simulink model "M12_addBlox"  (R2021a)
settings: Solver=ode45  StartTime=0.0  StopTime=10.0  RelTol=1e-3  EnableMultiTasking=on
undefined symbols (not defined in the file): magnitude, Tbit5_0
libraries: dspstat3 x4, simulink_extras x1, GeneralASKLib x1, commsink2 x1, NoiseLib_2021 x1
settings Model: Creator=Bornitz  LastModifiedBy=Bornitz
settings SolverCC: AlgebraicLoopSolver=TrustRegion
settings DataIOCC: LimitDataPoints=on  SaveFormat=Array
settings OptimizationCC: ExpressionDepthLimit=2147483647  LifeSpan=inf
settings DebuggingCC: SolverPrmCheckMsg=warning  StateNameClashWarn=warning  StrictBusMsg=ErrorOnBusTreatedAsVector  SFUnexpectedBacktrackingDiag=warning  SFNoUnconditionalDefaultTransitionDiag=warning  SFMachineParentedDataDiag=warning  ArithmeticOperatorsInVariantConditions=warning
settings HardwareCC: ProdBitPerPointer=32  ProdBitPerSizeT=32  ProdBitPerPtrDiffT=32  ProdLargestAtomicFloat=None  ProdIntDivRoundTo=Undefined  ProdEndianess=Unspecified  ProdWordSize=32  ProdHWDeviceType=32-bit Generic
settings ModelReferenceCC: PropagateSignalLabelsOutOfModel=off
settings SFSimCC: SimUseLocalCustomCode=off  SimParseCustomCode=off  CustomCodeUndefinedFunction=UseInterfaceOnly
settings RTWCC: RTWUseLocalCustomCode=off
settings CodeAppCC: StateflowObjectComments=on
settings GRTTargetCC: TargetLangStandard=C89/C90 (ANSI)  CombineOutputUpdateFcns=off  GRTInterface=on
settings ConfigComp: CovMetricSettings=dw  CovSaveCumulativeToWorkspaceVar=on  CovSaveSingleToWorkspaceVar=on  CovExternalEMLEnable=off  CovSFcnEnable=off

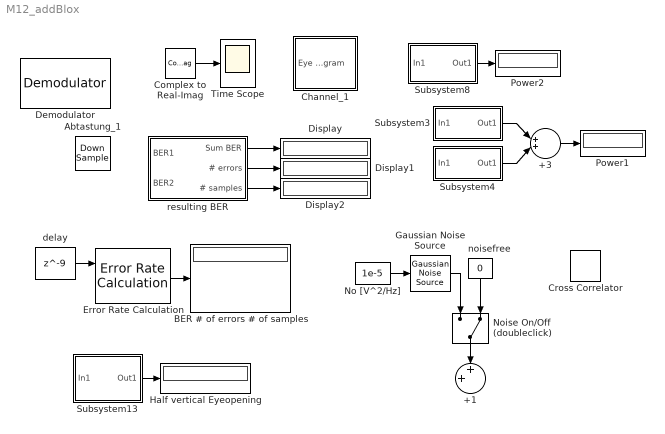
== system M12_addBlox ==
  " Power1" : Display
  " Power2" : Display
  +1 : Sum  Inputs=++|  SampleTime=Tbit5_0/16
  +3 : Sum  Inputs=||++||
  Abtastung_1 : DownSample  N=16  RateOptions=Allow multirate processing
  BER # of errors # of samples : Display
      settings: Format=short_e  Decimation=2
  Channel_1 : Subsystem
  Complex to Real-Imag : ComplexToRealImag  Output=Real
  Cross Correlator : simulink_extras/Additional Sinks/Cross Correlator  npts=100  HowOften=50  sampleT=0.0002
      settings: SourceProductBaseCode=SL
  Demodulator : GeneralASKLib/Demodulator  SystemSampleTime=-1  VariantActivationTime=update diagram  Latency=0  AutoFrameSizeCalculation=off
  Display : Display
      settings: Format=short_e
  Display1 : Display
  Display2 : Display
  Error Rate Calculation : commsink2/Error Rate Calculation  N=0  st_delay=100  cp_mode=Entire frame  subframe=1  PMode=Port  WsName=ErrorVec  RsMode2=off  stop=off  numErr=100  maxBits=1e6
  Gaussian Noise Source : NoiseLib_2021/Gaussian Noise Source  SystemSampleTime=-1  VariantActivationTime=update diagram  Latency=0  AutoFrameSizeCalculation=off
  Half vertical Eyeopening : Display
  No [V^2/Hz] : Constant  Value=1e-5
  Noise On/Off (doubleclick) : ManualSwitch  CurrentSetting=0
  Subsystem13 : Subsystem
      mask Display:
      | image('eye.bmp','center')
      | disp('\n\n\nEye Opening')
  Subsystem3 : Subsystem
      mask Display: disp('Power\n Measurement')
  Subsystem4 : Subsystem
      mask Display: disp('Power\n Measurement')
  Subsystem8 : Subsystem
      mask Display: disp('Power\n Measurement')
  Time Scope : Scope
  delay : Delay  DelayLength=9  InitialCondition=0  InputProcessing=Columns as channels (frame based)
  noisefree : Constant  Value=0
  resulting BER : Subsystem
  wires:
  Complex to Real-Imag/1 -> Time Scope/1
  Subsystem3/1(Out1) -> +3/1
  Subsystem4/1(Out1) -> +3/2
  +3/1 -> " Power1"/1
  Gaussian Noise Source/1 -> Noise On/Off (doubleclick)/1
  No [V^2/Hz]/1 -> Gaussian Noise Source/1
  noisefree/1 -> Noise On/Off (doubleclick)/2
  Noise On/Off (doubleclick)/1 -> +1/1
  Subsystem13/1(Out1) -> Half vertical Eyeopening/1
  delay/1 -> Error Rate Calculation/1
  Error Rate Calculation/1 -> BER # of errors # of samples/1
  resulting BER/3(# samples) -> Display2/1
  resulting BER/2(# errors) -> Display1/1
  resulting BER/1(Sum BER) -> Display/1
  Subsystem8/1(Out1) -> " Power2"/1

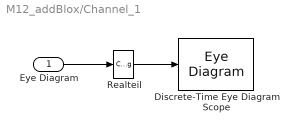
== system M12_addBlox/Channel_1 ==
  Eye Diagram : Inport
  Discrete-Time Eye Diagram Scope : EyeDiagram  Tag=EyeDiagram
  Realteil : ComplexToRealImag  Output=Real
  wires:
  Realteil/1 -> Discrete-Time Eye Diagram Scope/1
  Eye Diagram/1 -> Realteil/1

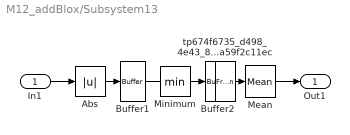
== system M12_addBlox/Subsystem13 ==
  In1 : Inport
  Abs : Abs
  Buffer1 : Buffer  N=20  V=4  OutputFrames=off
  Buffer2 : Buffer  N=200  V=4
  Mean : dspstat3/Mean  run=off  InputProcessing=Columns as channels (frame based)  reset_popup=None  directionMode=Each column  dimension=1  roiEnable=off  roiType=Rectangles  roiPortion=Entire ROI  roiOutput=Individual statistics for each ROI  roiFlag=off  roundingMode=Floor  overflowMode=off  outputDataTypeStr=Inherit: Same as accumulator  outputMin=[]  outputMax=[]  outputLastDataTypeStr=Inherit: Same as accumulator
  Minimum : MinMax
  tp674f6735_d498_4e43_822c_fba59f2c11ec : FrameConversion
  Out1 : Outport
  wires:
  tp674f6735_d498_4e43_822c_fba59f2c11ec/1 -> Minimum/1
  Buffer1/1 -> tp674f6735_d498_4e43_822c_fba59f2c11ec/1
  Mean/1 -> Out1/1
  In1/1 -> Abs/1
  Buffer2/1 -> Mean/1
  Minimum/1 -> Buffer2/1
  Abs/1 -> Buffer1/1

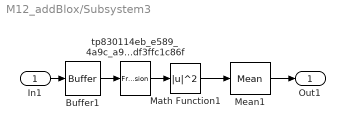
== system M12_addBlox/Subsystem3 ==
  In1 : Inport
  Buffer1 : Buffer  N=10*1024  OutputFrames=off
  Math Function1 : Math  Operator=magnitude^2  SignedPower=on  SaturateOnIntegerOverflow=on
  Mean1 : dspstat3/Mean  run=off  InputProcessing=Columns as channels (frame based)  reset_popup=None  directionMode=Each column  dimension=1  roiEnable=off  roiType=Rectangles  roiPortion=Entire ROI  roiOutput=Individual statistics for each ROI  roiFlag=off  roundingMode=Floor  overflowMode=off  outputDataTypeStr=Inherit: Same as accumulator  outputMin=[]  outputMax=[]  outputLastDataTypeStr=Inherit: Same as accumulator
  tp830114eb_e589_4a9c_a957_ddf3ffc1c86f : FrameConversion
  Out1 : Outport
  wires:
  tp830114eb_e589_4a9c_a957_ddf3ffc1c86f/1 -> Math Function1/1
  Buffer1/1 -> tp830114eb_e589_4a9c_a957_ddf3ffc1c86f/1
  Math Function1/1 -> Mean1/1
  In1/1 -> Buffer1/1
  Mean1/1 -> Out1/1

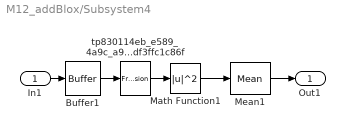
== system M12_addBlox/Subsystem4 ==
  In1 : Inport
  Buffer1 : Buffer  N=10*1024  OutputFrames=off
  Math Function1 : Math  Operator=magnitude^2  SignedPower=on  SaturateOnIntegerOverflow=on
  Mean1 : dspstat3/Mean  run=off  InputProcessing=Columns as channels (frame based)  reset_popup=None  directionMode=Each column  dimension=1  roiEnable=off  roiType=Rectangles  roiPortion=Entire ROI  roiOutput=Individual statistics for each ROI  roiFlag=off  roundingMode=Floor  overflowMode=off  outputDataTypeStr=Inherit: Same as accumulator  outputMin=[]  outputMax=[]  outputLastDataTypeStr=Inherit: Same as accumulator
  tp830114eb_e589_4a9c_a957_ddf3ffc1c86f : FrameConversion
  Out1 : Outport
  wires:
  tp830114eb_e589_4a9c_a957_ddf3ffc1c86f/1 -> Math Function1/1
  Buffer1/1 -> tp830114eb_e589_4a9c_a957_ddf3ffc1c86f/1
  Math Function1/1 -> Mean1/1
  In1/1 -> Buffer1/1
  Mean1/1 -> Out1/1

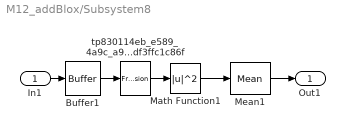
== system M12_addBlox/Subsystem8 ==
  In1 : Inport
  Buffer1 : Buffer  N=10*1024  OutputFrames=off
  Math Function1 : Math  Operator=magnitude^2  SignedPower=on  SaturateOnIntegerOverflow=on
  Mean1 : dspstat3/Mean  run=off  InputProcessing=Columns as channels (frame based)  reset_popup=None  directionMode=Each column  dimension=1  roiEnable=off  roiType=Rectangles  roiPortion=Entire ROI  roiOutput=Individual statistics for each ROI  roiFlag=off  roundingMode=Floor  overflowMode=off  outputDataTypeStr=Inherit: Same as accumulator  outputMin=[]  outputMax=[]  outputLastDataTypeStr=Inherit: Same as accumulator
  tp830114eb_e589_4a9c_a957_ddf3ffc1c86f : FrameConversion
  Out1 : Outport
  wires:
  tp830114eb_e589_4a9c_a957_ddf3ffc1c86f/1 -> Math Function1/1
  Buffer1/1 -> tp830114eb_e589_4a9c_a957_ddf3ffc1c86f/1
  Math Function1/1 -> Mean1/1
  In1/1 -> Buffer1/1
  Mean1/1 -> Out1/1

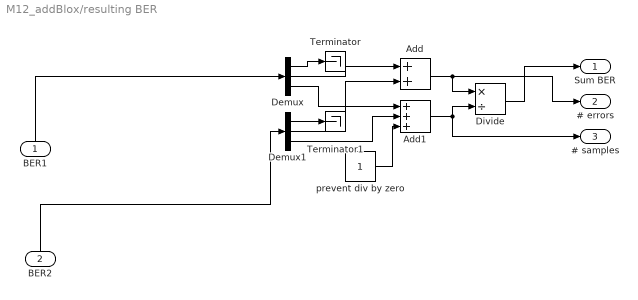
== system M12_addBlox/resulting BER ==
  BER1 : Inport
  BER2 : Inport  Port=2
  Add : Sum
  Add1 : Sum  Inputs=+++
  Demux : Demux  Outputs=3
  Demux1 : Demux  Outputs=3
  Divide : Product  Inputs=*/
  Terminator : Terminator
  Terminator1 : Terminator
  prevent div by zero : Constant
  Sum BER : Outport
  # errors : Outport  Port=2
  # samples : Outport  Port=3
  wires:
  BER1/1 -> Demux/1
  BER2/1 -> Demux1/1
  Demux/3 -> Add1/1
  Add1/1 -> # samples/1, Divide/2
  Demux/2 -> Add/1
  Add/1 -> # errors/1, Divide/1
  Demux1/3 -> Add1/2
  Demux1/2 -> Add/2
  Demux1/1 -> Terminator1/1
  Demux/1 -> Terminator/1
  Divide/1 -> Sum BER/1
  prevent div by zero/1 -> Add1/3
